simulink model "varSys"  (Simulink 7.6)
settings: Solver=ode45  StartTime=0.0  StopTime=10.0  RelTol=1e-3
PreLoadFcn:
  | var = 1;
  | varA = Simulink.Variant('var==1');
  | varB = Simulink.Variant('var==2');
settings Model: Creator=ajayaram  LastModifiedBy=ajayaram
settings OptimizationCC: InlineParams=on

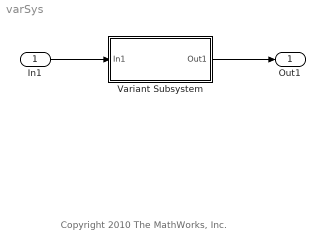
== system varSys ==
  note: Copyright 2010 The MathWorks, Inc.
  In1 : Inport
  Variant Subsystem : Subsystem  Variant=on
  Out1 : Outport
  wires:
  In1/1 -> Variant Subsystem/1(In1)
  Variant Subsystem/1(Out1) -> Out1/1

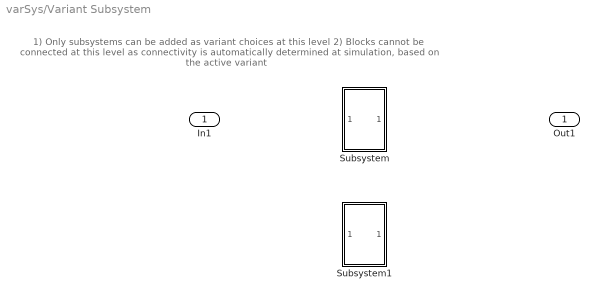
== system varSys/Variant Subsystem ==
  note: 1) Only subsystems can be added as variant choices at this level
      | 2) Blocks cannot be connected at this level as connectivity is
      | automatically determined at simulation, based on the active variant
  In1 : Inport
  Subsystem : Subsystem  TreatAsAtomicUnit=on  VariantObject=varA
  Subsystem1 : Subsystem  TreatAsAtomicUnit=on  VariantObject=varB
  Out1 : Outport

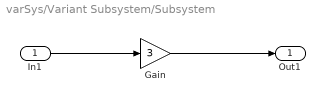
== system varSys/Variant Subsystem/Subsystem ==
  In1 : Inport
  Gain : Gain  Gain=3
  Out1 : Outport
  wires:
  Gain/1 -> Out1/1
  In1/1 -> Gain/1

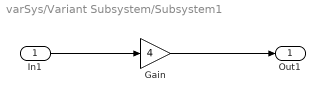
== system varSys/Variant Subsystem/Subsystem1 ==
  In1 : Inport
  Gain : Gain  Gain=4
  Out1 : Outport
  wires:
  In1/1 -> Gain/1
  Gain/1 -> Out1/1
